simulink model "pendulo"  (R2017a)
settings: Solver=ode45  StartTime=0  StopTime=190  MaxStep=.5  RelTol=1e-3  AbsTol=1e-6
libraries: fuzblock x1, simulink x1
settings Model: Creator=Adolfo  LastModifiedBy=bad
settings DataIOCC: ExternalInput=[]  InitialState=[]  LimitDataPoints=on  MaxDataPoints=10000  SaveFormat=Array  SignalLoggingSaveFormat=ModelDataLogs  SaveOutput=off  SaveTime=off
settings OptimizationCC: BlockReduction=off  BooleanDataType=off  ExpressionDepthLimit=2147483647  InitFltsAndDblsToZero=on  LifeSpan=inf
settings DebuggingCC: SaveWithParameterizedLinksMsg=none  UnderspecifiedInitializationDetection=Classic  MergeDetectMultiDrivingBlocksExec=none  SignalResolutionControl=TryResolveAllWithWarning  MultiTaskDSMMsg=warning  MultiTaskCondExecSysMsg=none  FcnCallInpInsideContextMsg=warning  StateNameClashWarn=warning  SFUnexpectedBacktrackingDiag=warning  SFNoUnconditionalDefaultTransitionDiag=warning  SFExecutionAtInitializationDiag=none
settings HardwareCC: ProdBitPerPointer=32  ProdBitPerSizeT=32  ProdBitPerPtrDiffT=32  ProdLargestAtomicFloat=None  ProdIntDivRoundTo=Undefined  ProdEndianess=Unspecified  ProdWordSize=32  ProdHWDeviceType=32-bit Generic  TargetUnknown=on
settings ModelReferenceCC: PropagateSignalLabelsOutOfModel=off
settings GRTTargetCC: TargetFcnLib=ansi_tfl_tmw.mat  TargetLangStandard=C89/C90 (ANSI)  CombineOutputUpdateFcns=off  GRTInterface=on
settings ConfigComp: CovMetricSettings=dw  CovHtmlReporting=on  CovSaveCumulativeToWorkspaceVar=on  CovSaveSingleToWorkspaceVar=on  CovExternalEMLEnable=off

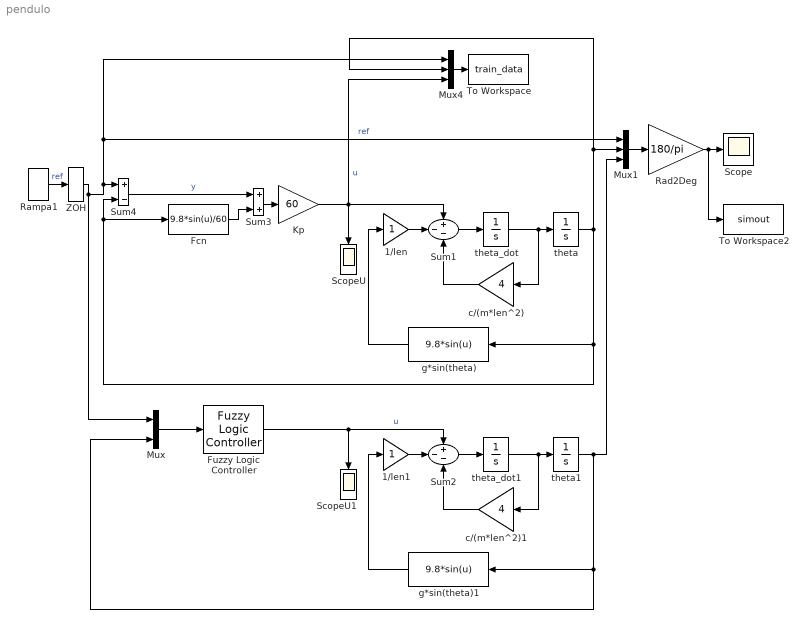
== system pendulo ==
  1/len : Gain  SaturateOnIntegerOverflow=on  OutDataTypeStr=Inherit: Same as input  ParamDataTypeStr=Inherit: Same as input
  1/len1 : Gain  SaturateOnIntegerOverflow=on  OutDataTypeStr=Inherit: Same as input  ParamDataTypeStr=Inherit: Same as input
  Fcn : Fcn  Expr=9.8*sin(u)/60
  Fuzzy Logic Controller : fuzblock/Fuzzy Logic  Controller  fis='anfis3.fis'
  Kp : Gain  Gain=60  SaturateOnIntegerOverflow=on  OutDataTypeStr=Inherit: Same as input  ParamDataTypeStr=Inherit: Same as input
  Mux : Mux  Inputs=2
  Mux1 : Mux  Inputs=3
  Mux4 : Mux  Inputs=3
  Rad2Deg : Gain  Gain=180/pi  SaturateOnIntegerOverflow=on  OutDataTypeStr=Inherit: Same as input  ParamDataTypeStr=Inherit: Same as input
  Rampa1 : simulink/Sources/Ramp  slope=pi/90  start=0  X0=-pi
  Scope : Scope
  ScopeU : Scope
  ScopeU1 : Scope
  Sum1 : Sum  Inputs=+--  SaturateOnIntegerOverflow=on  InputSameDT=on  OutDataTypeStr=Inherit: Same as first input
  Sum2 : Sum  Inputs=+--  SaturateOnIntegerOverflow=on  InputSameDT=on  OutDataTypeStr=Inherit: Same as first input
  Sum3 : Sum  SaturateOnIntegerOverflow=on  InputSameDT=on  OutDataTypeStr=Inherit: Same as first input
  Sum4 : Sum  Inputs=+-  SaturateOnIntegerOverflow=on  InputSameDT=on  OutDataTypeStr=Inherit: Same as first input
  To Workspace : ToWorkspace  VariableName=train_data  SaveFormat=Structure With Time  SampleTime=-1
  To Workspace2 : ToWorkspace  VariableName=simout  SaveFormat=Timeseries  SampleTime=-1
  ZOH : ZeroOrderHold  SampleTime=10
  c/(m*len^2) : Gain  Gain=4  SaturateOnIntegerOverflow=on  OutDataTypeStr=Inherit: Same as input  ParamDataTypeStr=Inherit: Same as input
  c/(m*len^2)1 : Gain  Gain=4  SaturateOnIntegerOverflow=on  OutDataTypeStr=Inherit: Same as input  ParamDataTypeStr=Inherit: Same as input
  g*sin(theta) : Fcn  Expr=9.8*sin(u)
  g*sin(theta)1 : Fcn  Expr=9.8*sin(u)
  theta : Integrator  InitialCondition=pi  UpperSaturationLimit=200  LowerSaturationLimit=-200
  theta1 : Integrator  InitialCondition=pi  UpperSaturationLimit=200  LowerSaturationLimit=-200
  theta_dot : Integrator  InitialCondition=-.1  UpperSaturationLimit=200  LowerSaturationLimit=-200
  theta_dot1 : Integrator  InitialCondition=-.1  UpperSaturationLimit=200  LowerSaturationLimit=-200
  wires:
  Sum1/1 -> theta_dot/1
  c/(m*len^2)/1 -> Sum1/3
  theta_dot/1 -> theta/1, c/(m*len^2)/1
  theta/1 -> g*sin(theta)/1, Fcn/1, Sum4/2, Mux4/2, Mux1/2
  1/len/1 -> Sum1/2
  g*sin(theta)/1 -> 1/len/1
  Sum4/1 -> Sum3/1  "y"
  Kp/1 -> Mux4/3, ScopeU/1, Sum1/1  "u"
  Mux1/1 -> Rad2Deg/1
  Rampa1/1 -> ZOH/1  "ref"
  Mux4/1 -> To Workspace/1
  Rad2Deg/1 -> To Workspace2/1, Scope/1
  1/len1/1 -> Sum2/2
  Fuzzy Logic Controller/1 -> ScopeU1/1, Sum2/1  "u"
  Sum2/1 -> theta_dot1/1
  g*sin(theta)1/1 -> 1/len1/1
  c/(m*len^2)1/1 -> Sum2/3
  theta1/1 -> Mux1/3, Mux/2, g*sin(theta)1/1
  theta_dot1/1 -> theta1/1, c/(m*len^2)1/1
  ZOH/1 -> Mux/1, Sum4/1, Mux4/1, Mux1/1  "ref"
  Mux/1 -> Fuzzy Logic Controller/1
  Sum3/1 -> Kp/1
  Fcn/1 -> Sum3/2
